simulink model "pendulum_1"  (R2020a)
settings: Solver=VariableStepAuto  StartTime=0.0  StopTime=10.0  MaxStep=0.01  RelTol=1e-3
libraries: simulink_extras x2
settings Model: EnablePacing=on  Creator=kiril_000  LastModifiedBy=kiril_000

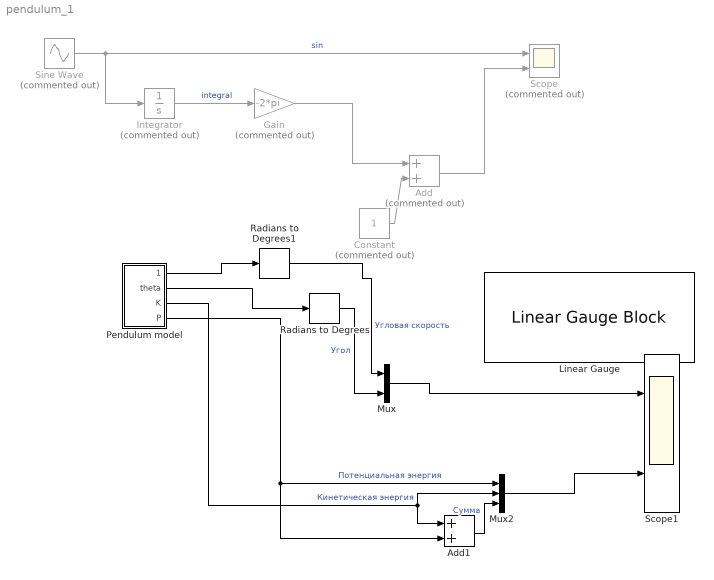
== system pendulum_1 ==
  Add : Sum  Commented=on
  Add1 : Sum
  Constant : Constant  Commented=on
  Gain : Gain  Commented=on  Gain=-2*pi
  Integrator : Integrator  Commented=on
  Linear Gauge : LinearGaugeBlock  ScaleMin=-90  ScaleMax=90
  Mux : Mux  Inputs=2
  Mux2 : Mux  Inputs=3
  Pendulum model : Subsystem  mask{m=1, l=1, g=9.8, b=0.5}
      mask prompts: m "Масса"; l "Длина"; g "Ускорение свободного падения"; b "Коэффициент вязкости"
      mask init:
      | I = m * l^2
  Radians to Degrees : simulink_extras/Transformations/Radians to Degrees
  Radians to Degrees1 : simulink_extras/Transformations/Radians to Degrees
  Scope : Scope  Commented=on  NumInputPorts=2
  Scope1 : Scope  NumInputPorts=2
  Sine Wave : Sin  Commented=on  Frequency=2*pi  SampleTime=0
  wires:
  Sine Wave/1 -> Integrator/1, Scope/1  "sin"
  Integrator/1 -> Gain/1  "integral"
  Gain/1 -> Add/1
  Constant/1 -> Add/2
  Add/1 -> Scope/2
  Radians to Degrees/1 -> Mux/2  "Угол"
  Pendulum model/2(theta) -> Radians to Degrees/1
  Pendulum model/1(dtheta) -> Radians to Degrees1/1
  Radians to Degrees1/1 -> Mux/1  "Угловая скорость"
  Mux/1 -> Scope1/1
  Pendulum model/4(P) -> Mux2/1, Add1/2  "Потенциальная энергия"
  Pendulum model/3(K) -> Mux2/2, Add1/1  "Кинетическая энергия"
  Add1/1 -> Mux2/3  "Сумма"
  Mux2/1 -> Scope1/2

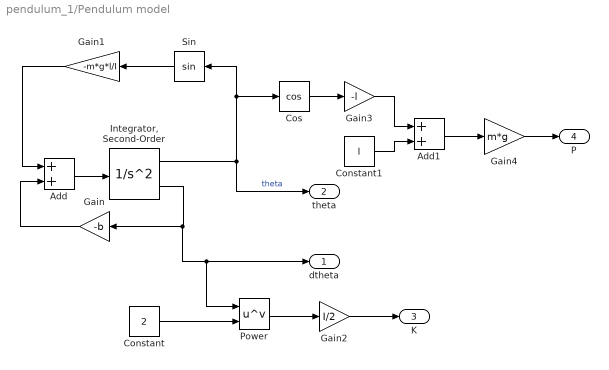
== system pendulum_1/Pendulum model ==
  Add : Sum
  Add1 : Sum
  Constant : Constant  Value=2
  Constant1 : Constant  Value=l
  Cos : Trigonometry  Operator=cos
  Gain : Gain  Gain=-b
  Gain1 : Gain  Gain=-m*g*l/I
  Gain2 : Gain  Gain=I/2
  Gain3 : Gain  Gain=-l
  Gain4 : Gain  Gain=m*g
  "Integrator, Second-Order" : SecondOrderIntegrator  ICX=deg2rad(15)
  Power : Math  Operator=pow  SaturateOnIntegerOverflow=on
  Sin : Trigonometry
  dtheta : Outport
  theta : Outport  Port=2
  K : Outport  Port=3
  P : Outport  Port=4
  wires:
  Sin/1 -> Gain1/1
  "Integrator, Second-Order"/2 -> Power/1, dtheta/1, Gain/1
  "Integrator, Second-Order"/1 -> Cos/1, Sin/1, theta/1  "theta"
  Gain1/1 -> Add/1
  Add/1 -> "Integrator, Second-Order"/1
  Gain/1 -> Add/2
  Constant/1 -> Power/2
  Power/1 -> Gain2/1
  Gain2/1 -> K/1
  Cos/1 -> Gain3/1
  Gain3/1 -> Add1/1
  Constant1/1 -> Add1/2
  Add1/1 -> Gain4/1
  Gain4/1 -> P/1
